simulink model "dcprojectnew"  (R2021a)
settings: Solver=VariableStepAuto  StartTime=0.0  StopTime=4e-3  RelTol=1e-3
InitFcn:
  | a = complex(ones(1,21));
undefined symbols (not defined in the file): magnitude
libraries: dspstat3 x3, commrflib2 x2, commfilt2 x2, dspmathops x1, simulink x1
settings Model: Creator=Utente  LastModifiedBy=Utente
settings DataIOCC: ExternalInput=a

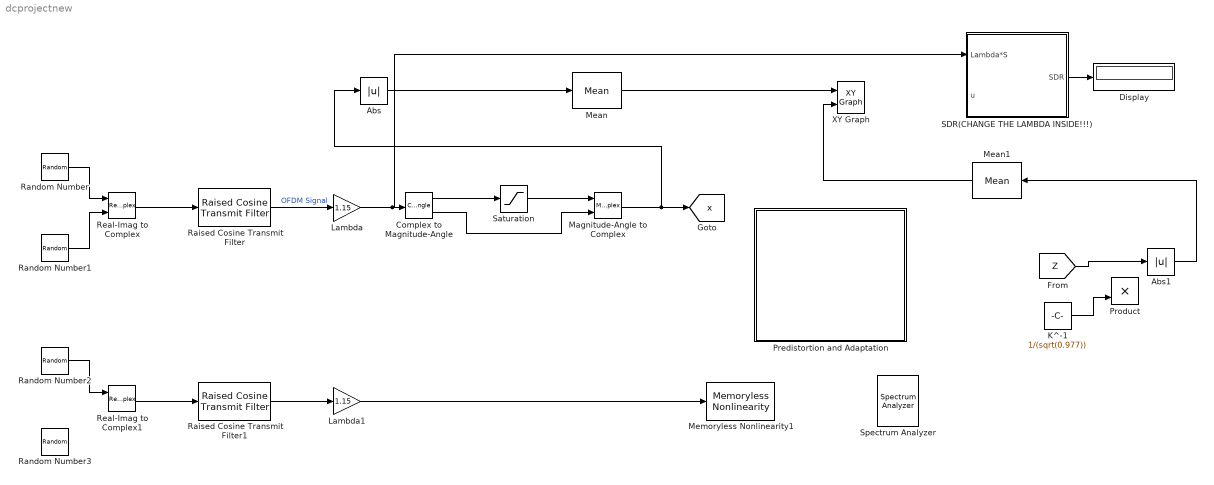
== system dcprojectnew ==
  Abs : Abs
  Abs1 : Abs
  Complex to Magnitude-Angle : ComplexToMagnitudeAngle
  Display : Display
  K^-1 : Constant  Value=1/(sqrt(0.977))
  Lambda : Gain  Gain=1.15
  Lambda1 : Gain  Gain=1.15
  Magnitude-Angle to Complex : MagnitudeAngleToComplex
  Mean : dspstat3/Mean  run=on  reset_popup=None  directionMode=Entire input  dimension=1  roiEnable=off  roiType=Rectangles  roiPortion=Entire ROI  roiOutput=Individual statistics for each ROI  roiFlag=off  roundingMode=Round  overflowMode=off  outputDataTypeStr=Inherit: Same as accumulator  outputMin=[]  outputMax=[]  outputLastDataTypeStr=Inherit: Same as accumulator
  Mean1 : dspstat3/Mean  run=on  reset_popup=None  directionMode=Entire input  dimension=1  roiEnable=off  roiType=Rectangles  roiPortion=Entire ROI  roiOutput=Individual statistics for each ROI  roiFlag=off  roundingMode=Round  overflowMode=off  outputDataTypeStr=Inherit: Same as accumulator  outputMin=[]  outputMax=[]  outputLastDataTypeStr=Inherit: Same as accumulator
  Memoryless Nonlinearity1 : commrflib2/Memoryless Nonlinearity  model_select=Rapp model  linGaindB=0  GindB=0  iip3=30  am2pm=10  LPwrLimAMPM=10  UPwrLimAMPM=inf  amam=[2.1587 1.1517]  ampm=[4.0033 9.1040]  x=[8.1081 1.5413 6.5202 -0.0718]  y=[4.6645 2.0965 10.88 -0.003]  p=2  GoutdB=0  vsat=1
      settings: SourceProductBaseCode=CM
  Predistortion and Adaptation : Subsystem
  Product : Product
  Raised Cosine Transmit Filter : commfilt2/Raised Cosine Transmit Filter  filtType=Square root  R=0.2  filtSpan=80  N=8  filterGain=1  RateOptions=Allow multirate processing  framing=Mute  checkCoeff=off  variableName=rcTxFilt  checkGain=Normalized  sampMode=Mute  saveAsFlag=0  currentFiltSpan=10  D=(10)/2  launchFVT=on  roundingMode=Floor  overflowMode=off  coeffDataTypeStr=Inherit: Same word length as input  coeffMin=[]  coeffMax=[]  coeffLastDataTypeStr=Inherit: Same word length as input  outputDataTypeStr=Inherit: Same as accumulator  outputMin=[]  outputMax=[]  outputLastDataTypeStr=Inherit: Same as accumulator
  Raised Cosine Transmit Filter1 : commfilt2/Raised Cosine Transmit Filter  filtType=Square root  R=0.2  filtSpan=80  N=8  filterGain=1  RateOptions=Allow multirate processing  framing=Mute  checkCoeff=off  variableName=rcTxFilt1  checkGain=Normalized  sampMode=Mute  saveAsFlag=0  currentFiltSpan=10  D=(10)/2  launchFVT=on  roundingMode=Floor  overflowMode=off  coeffDataTypeStr=Inherit: Same word length as input  coeffMin=[]  coeffMax=[]  coeffLastDataTypeStr=Inherit: Same word length as input  outputDataTypeStr=Inherit: Same as accumulator  outputMin=[]  outputMax=[]  outputLastDataTypeStr=Inherit: Same as accumulator
  Random Number : RandomNumber  Variance=100  Seed=1  SampleTime=0.0000001
  Random Number1 : RandomNumber  Variance=100  Seed=1  SampleTime=0.0000001
  Random Number2 : RandomNumber  SampleTime=0.0000001
  Random Number3 : RandomNumber  Variance=0.5  Seed=1  SampleTime=0.0000001
  Real-Imag to Complex : RealImagToComplex
  Real-Imag to Complex1 : RealImagToComplex
  SDR(CHANGE THE LAMBDA INSIDE!!!) : Subsystem
  Saturation : Saturate  UpperLimit=1  LowerLimit=0
  Spectrum Analyzer : SpectrumAnalyzer
  XY Graph : simulink/Sinks/XY Graph  xmin=0  xmax=2  ymin=0  ymax=2  st=-1
  tag scope: x=global
  wires:
  Random Number/1 -> Real-Imag to Complex/1
  Real-Imag to Complex/1 -> Raised Cosine Transmit Filter/1
  Raised Cosine Transmit Filter/1 -> Lambda/1  "OFDM Signal"
  Lambda/1 -> SDR(CHANGE THE LAMBDA INSIDE!!!)/1(Lambda*S), Complex to Magnitude-Angle/1
  Complex to Magnitude-Angle/1 -> Saturation/1
  Saturation/1 -> Magnitude-Angle to Complex/1
  Complex to Magnitude-Angle/2 -> Magnitude-Angle to Complex/2
  Magnitude-Angle to Complex/1 -> Abs/1, [x]
  Real-Imag to Complex1/1 -> Raised Cosine Transmit Filter1/1
  Raised Cosine Transmit Filter1/1 -> Lambda1/1
  Random Number2/1 -> Real-Imag to Complex1/1
  Lambda1/1 -> Memoryless Nonlinearity1/1
  K^-1/1 -> Product/2
  Random Number1/1 -> Real-Imag to Complex/2
  [Z] -> Abs1/1
  SDR(CHANGE THE LAMBDA INSIDE!!!)/1(SDR) -> Display/1
  Abs/1 -> Mean/1
  Abs1/1 -> Mean1/1
  Mean1/1 -> XY Graph/2
  Mean/1 -> XY Graph/1

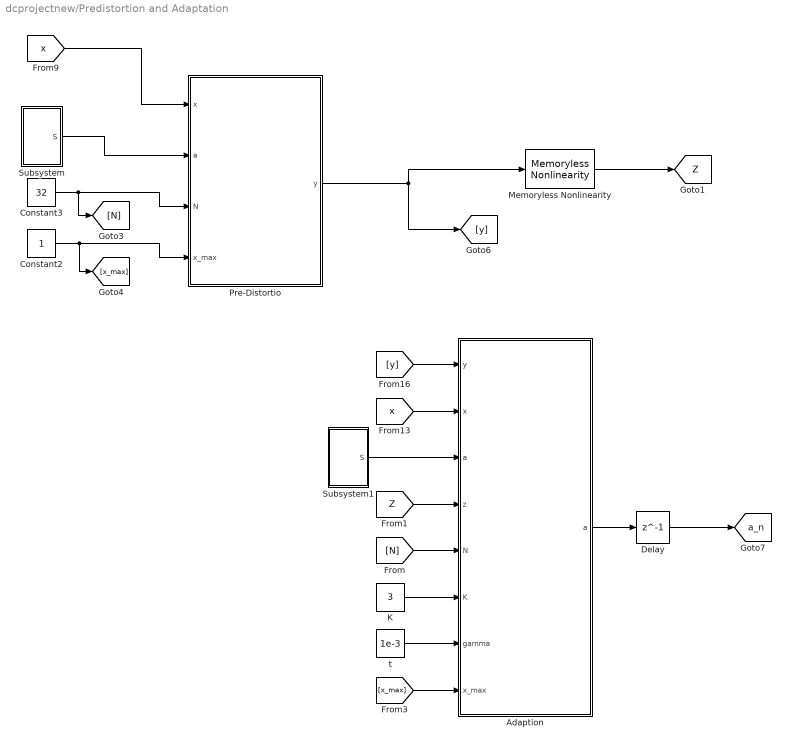
== system dcprojectnew/Predistortion and Adaptation ==
  "Adaption " : MATLAB Function  TreatAsAtomicUnit=on
  Constant2 : Constant
  Constant3 : Constant  Value=32
  Delay : Delay  DelayLength=1  InitialCondition=0
  K : Constant  Value=3
  Memoryless Nonlinearity : commrflib2/Memoryless Nonlinearity  model_select=Rapp model  linGaindB=0  GindB=0  iip3=30  am2pm=10  LPwrLimAMPM=10  UPwrLimAMPM=inf  amam=[2.1587 1.1517]  ampm=[4.0033 9.1040]  x=[8.1081 1.5413 6.5202 -0.0718]  y=[4.6645 2.0965 10.88 -0.003]  p=20  GoutdB=0  vsat=1
      settings: SourceProductBaseCode=CM
  Pre-Distortio : MATLAB Function  TreatAsAtomicUnit=on
  Subsystem : Subsystem
  Subsystem1 : Subsystem
  t : Constant  Value=1e-3
  tag scope: Z=global, a_n=global
  wires:
  [x] -> "Adaption "/2(x)
  "Adaption "/1(a) -> Delay/1
  [x] -> Pre-Distortio/1(x)
  Delay/1 -> [a_n]
  [x_max] -> "Adaption "/8(x_max)
  Constant3/1 -> Pre-Distortio/3(N), [N]
  Pre-Distortio/1(y) -> Memoryless Nonlinearity/1, [y]
  [Z] -> "Adaption "/4(z)
  [y] -> "Adaption "/1(y)
  [N] -> "Adaption "/5(N)
  t/1 -> "Adaption "/7(gamma)
  Constant2/1 -> [x_max], Pre-Distortio/4(x_max)
  K/1 -> "Adaption "/6(K)
  Memoryless Nonlinearity/1 -> [Z]
  Subsystem/1(S) -> Pre-Distortio/2(a)
  Subsystem1/1(S) -> "Adaption "/3("a ")

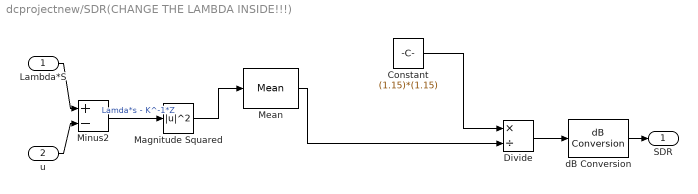
== system dcprojectnew/SDR(CHANGE THE LAMBDA INSIDE!!!) ==
  Lambda*S : Inport
  u : Inport  Port=2
  Constant : Constant  Value=(1.15)*(1.15)
  Divide : Product  Inputs=*/
  Magnitude Squared : Math  Operator=magnitude^2  OutputSignalType=real  SaturateOnIntegerOverflow=on
  Mean : dspstat3/Mean  run=on  reset_popup=None  directionMode=Entire input  dimension=1  roiEnable=off  roiType=Rectangles  roiPortion=Entire ROI  roiOutput=Individual statistics for each ROI  roiFlag=off  roundingMode=Round  overflowMode=off  outputDataTypeStr=Inherit: Same as accumulator  outputMin=[]  outputMax=[]  outputLastDataTypeStr=Inherit: Same as accumulator
  Minus2 : Sum  Inputs=+-
  dB Conversion : dspmathops/dB Conversion  dBtype=dB  intype=Power  R=1  fuzz=off
  SDR : Outport
  wires:
  Mean/1 -> Divide/2
  Constant/1 -> Divide/1
  dB Conversion/1 -> SDR/1
  Lambda*S/1 -> Minus2/1
  Magnitude Squared/1 -> Mean/1
  Minus2/1 -> Magnitude Squared/1  "Lamda*s - K^-1*Z"
  Divide/1 -> dB Conversion/1
  u/1 -> Minus2/2

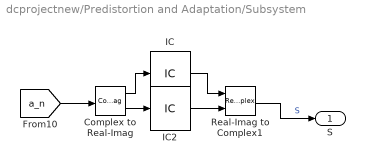
== system dcprojectnew/Predistortion and Adaptation/Subsystem ==
  Complex to Real-Imag : ComplexToRealImag
  IC : InitialCondition  Value=ones(1,33)
  IC2 : InitialCondition  Value=zeros(1,33)
  Real-Imag to Complex1 : RealImagToComplex
  S : Outport
  wires:
  Complex to Real-Imag/2 -> IC2/1
  IC2/1 -> Real-Imag to Complex1/2
  [a_n] -> Complex to Real-Imag/1
  IC/1 -> Real-Imag to Complex1/1
  Complex to Real-Imag/1 -> IC/1
  Real-Imag to Complex1/1 -> S/1  "S"

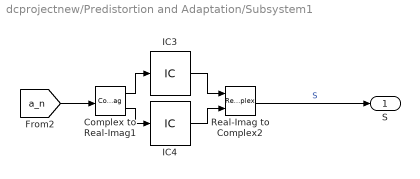
== system dcprojectnew/Predistortion and Adaptation/Subsystem1 ==
  Complex to Real-Imag1 : ComplexToRealImag
  IC3 : InitialCondition  Value=ones(1,33)
  IC4 : InitialCondition  Value=zeros(1,33)
  Real-Imag to Complex2 : RealImagToComplex
  S : Outport
  wires:
  IC4/1 -> Real-Imag to Complex2/2
  [a_n] -> Complex to Real-Imag1/1
  Real-Imag to Complex2/1 -> S/1  "S"
  Complex to Real-Imag1/2 -> IC4/1
  IC3/1 -> Real-Imag to Complex2/1
  Complex to Real-Imag1/1 -> IC3/1

== matlab function dcprojectnew/Predistortion and Adaptation/Pre-Distortio ==
  data: x input; y output size=1; a input; N input; x_max input
function y  = predistortion(x,a,N,x_max)
    %Interval detection
    delta = abs(x_max) / (2*N); 
    % All intervals
    I = [delta*2:delta*2:x_max inf];
    % Find the Parameter Index where the abs(x) falls
    n = 1:(N+1);
    n = n(abs(x) < I);
    n = n(1);
    % Piecewise Linear Interpolation
    P_x = ((abs(x) - (2*n-1)*delta) * (a(min(n+1,N+1)) - a(n)) / (2*delta)) + ((a(min(n+1,N+1)) + a(n)) / 2);
    % Output
    y_old = complex( x * P_x);
    y = y_old;
end

== matlab function dcprojectnew/Predistortion and Adaptation/Adaption  ==
  data: y input; x input; a input; a output; z input; N input; K input; gamma input; x_max input
function a = Adaption(y, x, a, z, N, K, gamma, x_max)
    
    %Re-do the same because of causality of the first initialization
    delta = abs(x_max) / (2*N);
    % All Intervals
    I = [delta:delta*2:x_max inf];
    n = 1:(N+1);
    n = n(abs(x) < I);
    n = n(1);
    % Update Coefficients
    a(n) = (a(n) - gamma * (z - K * x) * conj(z) / conj(y) * conj(x)); 
end
